simulink model "LQG_Sim"  (R2018b)
settings: Solver=FixedStepAuto  StartTime=0.0  StopTime=10  RelTol=1e-3
values from neighbouring files (symbols this model uses):
  Bw = eye(n)    [LQG_Sim.m]
  K = K_hat(1:m,1:n)    [LQG_Sim.m]    (also in LQR_PI_Sim.m; LQR_P_Sim.m = lqr(A,B,Q,R))
  Ki = -K_hat(1:m,n+1:n+p)    [LQG_Sim.m]    (also in LQR_PI_Sim.m)
  n = 4    [LQG_Sim.m]    (also in LQR_PI_Sim.m)
  p = 2    [LQG_Sim.m]    (also in LQR_PI_Sim.m)
  Re = diag(ones(size(C,1)))    [LQG_Sim.m]
undefined symbols (not defined in the file or in its folder): A, B, C, Continuous, D, Time
libraries: simulink_extras x2, ctrlSharedLib x1
settings Model: Creator=smiah-admin  LastModifiedBy=gjaniak

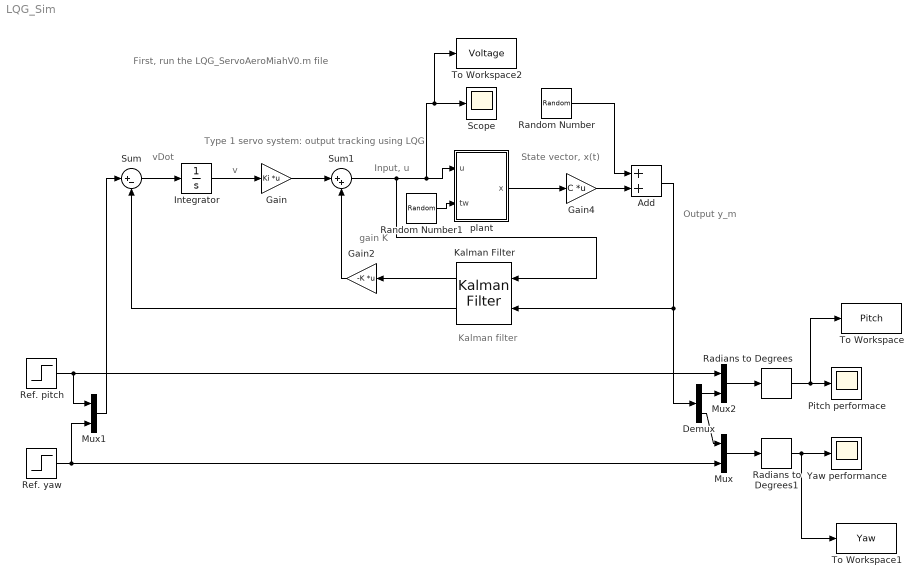
== system LQG_Sim ==
  note: Kalman filter
  note: State vector, x(t)
  note: Input, u
  note: First, run the LQG_ServoAeroMiahV0.m file
  note: Type 1 servo system: output tracking using LQG
  note: Output y_m
  note: vDot
  note: gain K
  note: v
  Add : Sum
  Demux : Demux  Outputs=2
  Gain : Gain  Gain=Ki  Multiplication=Matrix(K*u)
  Gain2 : Gain  Gain=-K  Multiplication=Matrix(K*u)
  Gain4 : Gain  Gain=C  Multiplication=Matrix(K*u)
  Integrator : Integrator
  Kalman Filter : ctrlSharedLib/Kalman Filter  TimeDomain=Continuous-Time  UseCurrentEstimator=on  ModelSource=Individual A, B, C, D matrices  ModelSourceVariable=ss(0.95,1,1,0,1)  A=A  B=B  C=C  D=D  NumberOfStates=1  NumberOfInputs=1  NumberOfOutputs=1  InitialEstimateSource=Dialog  X0=0  P0=10  UseK=off  UseGH=off  NumberOfProcessNoiseInputs=1  G=1  TimeInvariantG=on  H=0  TimeInvariantH=on  Q=Qe  TimeInvariantQ=on  R=Re  TimeInvariantR=on  N=0  TimeInvariantN=on  AddInputPort=on  AddEnablePort=off  OutputEstimatedY=on  OutputP=off  Ts=-1
      settings: SourceProductBaseCode=CT
  Mux : Mux  Inputs=2
  Mux1 : Mux  Inputs=2
  Mux2 : Mux  Inputs=2
  Pitch performace : Scope
  Radians to Degrees : simulink_extras/Transformations/Radians to Degrees
  Radians to Degrees1 : simulink_extras/Transformations/Radians to Degrees
  Random Number : RandomNumber  Variance=1e-8*(ones(p,1))  SampleTime=0.1
  Random Number1 : RandomNumber  Variance=1e-8*(ones(n,1))  SampleTime=0.1
  "Ref. pitch " : Step  Time=0  After=45*pi/180  SampleTime=.01
  Ref. yaw : Step  Time=0  After=180*pi/180  SampleTime=0.01
  Scope : Scope
  Sum : Sum  Inputs=|+-
  Sum1 : Sum  Inputs=|++
  To Workspace : ToWorkspace  VariableName=Pitch  SaveFormat=Structure With Time  SampleTime=-1
  To Workspace1 : ToWorkspace  VariableName=Yaw  SaveFormat=Structure With Time  SampleTime=-1
  To Workspace2 : ToWorkspace  VariableName=Voltage  SaveFormat=Structure With Time  SampleTime=-1
  "Yaw performance " : Scope
  plant : Subsystem
      mask help: Plant
  wires:
  Gain2/1 -> Sum1/2
  Gain/1 -> Sum1/1
  Sum/1 -> Integrator/1
  Integrator/1 -> Gain/1
  Sum1/1 -> Kalman Filter/1, To Workspace2/1, Scope/1, plant/1(u)
  plant/1(x) -> Gain4/1
  "Ref. pitch "/1 -> Mux2/1, Mux1/1
  Ref. yaw/1 -> Mux1/2, Mux/2
  Mux1/1 -> Sum/1
  Demux/2 -> Mux/1
  Demux/1 -> Mux2/2
  Kalman Filter/1 -> Gain2/1
  Kalman Filter/2 -> Sum/2
  Random Number1/1 -> plant/2(tw)
  Gain4/1 -> Add/2
  Random Number/1 -> Add/1
  Add/1 -> Demux/1, Kalman Filter/2
  Mux2/1 -> Radians to Degrees/1
  Radians to Degrees/1 -> To Workspace/1, Pitch performace/1
  Mux/1 -> Radians to Degrees1/1
  Radians to Degrees1/1 -> "Yaw performance "/1, To Workspace1/1

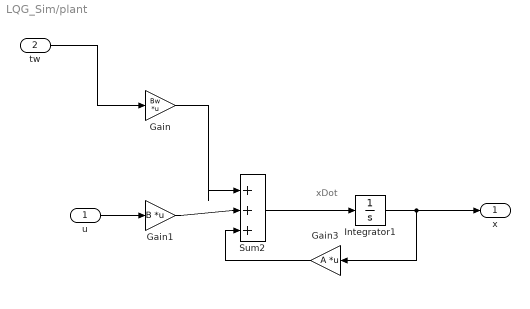
== system LQG_Sim/plant ==
  note: xDot
  u : Inport
  tw : Inport  Port=2
  Gain : Gain  Gain=Bw  Multiplication=Matrix(K*u)
  Gain1 : Gain  Gain=B  Multiplication=Matrix(K*u)
  Gain3 : Gain  Gain=A  Multiplication=Matrix(K*u)
  Integrator1 : Integrator
  Sum2 : Sum  Inputs=|+++
  x : Outport
  wires:
  Integrator1/1 -> Gain3/1, x/1
  Sum2/1 -> Integrator1/1
  u/1 -> Gain1/1
  Gain3/1 -> Sum2/3
  Gain1/1 -> Sum2/2
  tw/1 -> Gain/1
  Gain/1 -> Sum2/1
